simulink library "nodePosToLinkPos_ul"  (R2022a)
settings: Solver=VariableStepAuto  StartTime=0.0  StopTime=10.0  RelTol=1e-3
libraries: matrix_library x2
settings Model: Creator=James Reed  LastModifiedBy=lhill8
settings SolverCC: AlgebraicLoopSolver=TrustRegion
settings DebuggingCC: UnconnectedInputMsg=warning  UnconnectedOutputMsg=warning  UnconnectedLineMsg=warning  SFMachineParentedDataDiag=warning  ArithmeticOperatorsInVariantConditions=warning
settings SFSimCC: CustomCodeUndefinedFunction=UseInterfaceOnly

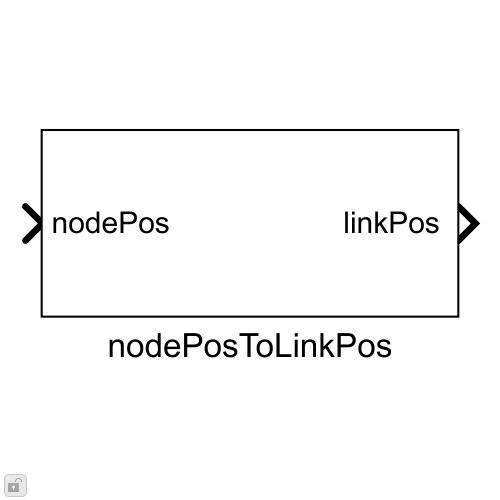
[thumbnail: Simulink's stored preview of the top-level diagram]
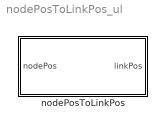
== system nodePosToLinkPos_ul ==
  nodePosToLinkPos : Subsystem

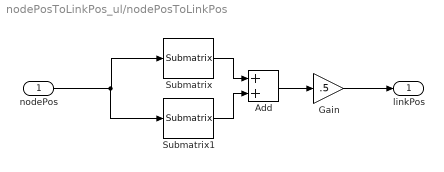
== system nodePosToLinkPos_ul/nodePosToLinkPos ==
  "nodePos " : Inport
  Add : Sum
  Gain : Gain  Gain=.5
  Submatrix : matrix_library/Submatrix  RowSpan=All rows  RowStartMode=First  RowStartIndex=1  RowEndMode=Last  RowEndIndex=1  ColSpan=Range of columns  ColStartMode=First  ColStartIndex=1  ColEndMode=Offset from last  ColEndIndex=1
      settings: SourceProductBaseCode=SL
  Submatrix1 : matrix_library/Submatrix  RowSpan=All rows  RowStartMode=First  RowStartIndex=1  RowEndMode=Last  RowEndIndex=1  ColSpan=Range of columns  ColStartMode=Index  ColStartIndex=2  ColEndMode=Last  ColEndIndex=1
      settings: SourceProductBaseCode=SL
  "linkPos " : Outport  VectorParamsAs1DForOutWhenUnconnected=off
  wires:
  "nodePos "/1 -> Submatrix1/1, Submatrix/1
  Gain/1 -> "linkPos "/1
  Add/1 -> Gain/1
  Submatrix/1 -> Add/1
  Submatrix1/1 -> Add/2
